simulink model "M10B39_V2"  (R2025a)
settings: Solver=ode23tb  StartTime=0.0  StopTime=1000  FixedStep=0.001  RelTol=1e-3  EnableMultiTasking=on
InitFcn:
  | clear;
  | initAll_V2;
  | %set_param('M10B39/Python2Sim','value','zeros(1,16)');
values from neighbouring files (symbols this model uses):
  acom = 100    [initAll.m]    (also in initAll_V2.m)
  bcom = 50    [initAll.m]    (also in initAll_V2.m)
  commun = 0*commun    [initAll.m]    (also in initAll_V2.m)
  DataDelay = 0.0*DataDelay    [initAll.m]    (also in initAll_V2.m)
  fB = 50    [initAll.m]    (also in initAll_V2.m)
  Geninit = Generator_init(opdata,SynMach_in_gidx)    [initAll.m]    (also in initAll_V2.m)
  lam = 100    [initAll.m]    (also in initAll_V2.m)
  loadnode = 31    [initAll_V2.m]
  loadsize = 16.2714    [initAll_V2.m]
  SgridB = 100    [initAll.m]    (also in initAll_V2.m)
  wB = 2*pi*fB    (= 314.159265359)    [initAll.m]    (also in initAll_V2.m)
undefined symbols (not defined in the file or in its folder): AVm0, c1, c2, c3, c4, c5, c6, cp_nom, ESinit, lambda_nom, P_wind_base, Pelec_base, Pnom, Windinit, YY_load
libraries: spsBistableLib x13, simulink_extras x5, powerlib_meascontrol x2, simulink x1
(part 4 of 11)

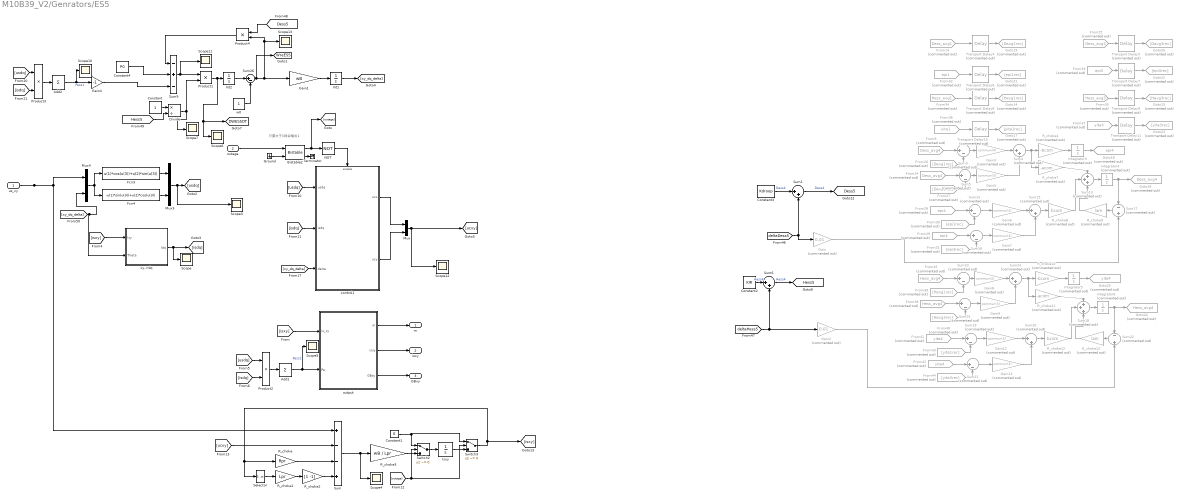
== system M10B39_V2/Genrators/ES5 ==
  note: 只要大于0就会输出1
  us_xy : Inport
  outage : Inport  Port=2
  " control1" : Subsystem
  Add1 : Sum  Inputs=+
  Add2 : Sum  Inputs=+
  Bistable2 : spsBistableLib/Bistable  Qpriority=Set  ic=0  Ts=0
      settings: LibrarySourceBlock=sps_lib/Control/Bistable
  Constant : Constant
  Constant1 : Constant  Value=0
  Constant2 : Constant  Value=KIR
  Constant3 : Constant  Value=Kdroop
  Constant4 : Constant  Value=P0
  Divide : Product  Inputs=*/
  Fcn3 : Fcn  Expr=u(1)*cos(u(3))+u(2)*sin(u(3))
  Fcn4 : Fcn  Expr=-u(1)*sin(u(3))+u(2)*cos(u(3))
  From14 : From  Commented=on  GotoTag=Dess_avg1  TagVisibility=global
  From24 : From  Commented=on  GotoTag=Dess_avg4  TagVisibility=global
  From25 : From  Commented=on  GotoTag=Dess_avg3  TagVisibility=global
  From26 : From  Commented=on  GotoTag=Davg1rec
  From27 : From  Commented=on  GotoTag=Davg3rec
  From28 : From  Commented=on  GotoTag=epi4  TagVisibility=global
  From29 : From  Commented=on  GotoTag=epi4  TagVisibility=global
  From30 : From  Commented=on  GotoTag=epi1rec
  From31 : From  Commented=on  GotoTag=epi3rec
  From32 : From  Commented=on  GotoTag=epi1  TagVisibility=global
  From33 : From  Commented=on  GotoTag=epi3  TagVisibility=global
  From34 : From  Commented=on  GotoTag=Hess_avg1  TagVisibility=global
  From35 : From  Commented=on  GotoTag=Hess_avg3  TagVisibility=global
  From36 : From  Commented=on  GotoTag=yita1  TagVisibility=global
  From37 : From  Commented=on  GotoTag=yita3  TagVisibility=global
  From38 : From  Commented=on  GotoTag=Hess_avg4  TagVisibility=global
  From39 : From  Commented=on  GotoTag=Havg1rec
  From40 : From  Commented=on  GotoTag=Havg3rec
  From41 : From  Commented=on  GotoTag=yita4  TagVisibility=global
  From42 : From  Commented=on  GotoTag=yita4  TagVisibility=global
  From43 : From  Commented=on  GotoTag=yita1rec
  From44 : From  Commented=on  GotoTag=yita3rec
  From45 : From  Commented=on  GotoTag=Hess_avg4  TagVisibility=global
  From9 : From  Commented=on  GotoTag=Dess_avg4  TagVisibility=global
  Gain : Gain  Commented=on  Gain=0.01
  Gain1 : Gain  Gain=wB  SaturateOnIntegerOverflow=on  OutDataTypeStr=Inherit: Same as input  ParamDataTypeStr=Inherit: Same as input
  Gain{3,6,8,12} (4 alike) : Gain  Commented=on  Gain=commun(4)
  Gain{5,7,9,13} (4 alike) : Gain  Commented=on  Gain=commun(3)
  Gain2 : Gain  Commented=on  Gain=0.01
  Gain4 : Gain  Gain=-1
  Goto14 : Goto  Commented=on  GotoTag=Havg1rec
  Goto15 : Goto  Commented=on  GotoTag=Havg3rec
  Goto16 : Goto  Commented=on  GotoTag=Dess_avg4  TagVisibility=global
  Goto17 : Goto  Commented=on  GotoTag=yita1rec
  Goto18 : Goto  Commented=on  GotoTag=epi4  TagVisibility=global
  Goto19 : Goto  Commented=on  GotoTag=Davg1rec
  Goto20 : Goto  Commented=on  GotoTag=Davg3rec
  Goto21 : Goto  Commented=on  GotoTag=epi1rec
  Goto22 : Goto  Commented=on  GotoTag=epi3rec
  Goto23 : Goto  Commented=on  GotoTag=yita3rec
  Goto24 : Goto  Commented=on  GotoTag=Hess_avg4  TagVisibility=global
  Goto25 : Goto  Commented=on  GotoTag=yita4  TagVisibility=global
  Ground : Ground
  Int1 : Integrator  InitialCondition=Dels_hvdc
  Int2 : Integrator  InitialCondition=1
  Integrator{3..6} (4 alike) : Integrator  Commented=on
  Isxy : Integrator  InitialCondition=[Is_xA_0 Is_yA_0]
  Mux : Mux  Inputs=2
  Mux3 : Mux  Inputs=2
  Mux4 : Mux  Inputs=2
  NOT : Logic  Operator=NOT  AllPortsSameDT=off  OutDataTypeStr=boolean
  Product1 : Product
  Product2 : Product  RndMeth=Zero
  Product3 : Product  RndMeth=Zero
  Product4 : Product
  R_choke : Gain  Gain=Rpr  SaturateOnIntegerOverflow=on  OutDataTypeStr=Inherit: Same as input  ParamDataTypeStr=Inherit: Same as input
  R_choke1 : Gain  Gain=Lpr  SaturateOnIntegerOverflow=on  OutDataTypeStr=Inherit: Same as input  ParamDataTypeStr=Inherit: Same as input
  R_choke10 : Gain  Commented=on  Gain=-bcom  SaturateOnIntegerOverflow=on  OutDataTypeStr=Inherit: Same as input  ParamDataTypeStr=Inherit: Same as input
  R_choke11 : Gain  Commented=on  Gain=-acom  SaturateOnIntegerOverflow=on  OutDataTypeStr=Inherit: Same as input  ParamDataTypeStr=Inherit: Same as input
  R_choke12 : Gain  Commented=on  Gain=bcom  SaturateOnIntegerOverflow=on  OutDataTypeStr=Inherit: Same as input  ParamDataTypeStr=Inherit: Same as input
  R_choke13 : Gain  Commented=on  Gain=lam  SaturateOnIntegerOverflow=on  OutDataTypeStr=Inherit: Same as input  ParamDataTypeStr=Inherit: Same as input
  R_choke2 : Gain  Gain=[1 -1]  SaturateOnIntegerOverflow=on  OutDataTypeStr=Inherit: Same as input  ParamDataTypeStr=Inherit: Same as input
  R_choke3 : Gain  Gain=wB / Lpr  SaturateOnIntegerOverflow=on  OutDataTypeStr=Inherit: Same as input  ParamDataTypeStr=Inherit: Same as input
  R_choke4 : Gain  Commented=on  Gain=-bcom  SaturateOnIntegerOverflow=on  OutDataTypeStr=Inherit: Same as input  ParamDataTypeStr=Inherit: Same as input
  R_choke7 : Gain  Commented=on  Gain=-acom  SaturateOnIntegerOverflow=on  OutDataTypeStr=Inherit: Same as input  ParamDataTypeStr=Inherit: Same as input
  R_choke8 : Gain  Commented=on  Gain=bcom  SaturateOnIntegerOverflow=on  OutDataTypeStr=Inherit: Same as input  ParamDataTypeStr=Inherit: Same as input
  R_choke9 : Gain  Commented=on  Gain=lam  SaturateOnIntegerOverflow=on  OutDataTypeStr=Inherit: Same as input  ParamDataTypeStr=Inherit: Same as input
  Scope{,3..7,10..13} (10 alike) : Scope
      Scope settings: ActiveDisplayYMinimum=-0.0194  ActiveDisplayYMaximum=0.04689
      Scope10 settings: ActiveDisplayYMinimum=-6.46308  ActiveDisplayYMaximum=-6.45084
      Scope11 settings: ActiveDisplayYMinimum=-0.1125  ActiveDisplayYMaximum=0.0125  DataLoggingVariableName=ScopeData2
      Scope12 settings: ActiveDisplayYMinimum=0.46883  ActiveDisplayYMaximum=1.25548  DataLoggingVariableName=ScopeData3
      Scope13 settings: ActiveDisplayYMinimum=-0.00656  ActiveDisplayYMaximum=0.05904  DataLoggingVariableName=ScopeData4
      Scope3 settings: ActiveDisplayYMinimum=-0.12696  ActiveDisplayYMaximum=1.14248
      Scope4 settings: ActiveDisplayYMinimum=-2.8E-5  ActiveDisplayYMaximum=2.4E-5  DataLoggingVariableName=ScopeData5
      Scope5 settings: ActiveDisplayYMinimum=-0.00823  ActiveDisplayYMaximum=0.07404  DataLoggingVariableName=ScopeData7
      Scope6 settings: ActiveDisplayYMinimum=-4.9E-5  ActiveDisplayYMaximum=-0  DataLoggingVariableName=ScopeData4
      Scope7 settings: ActiveDisplayYMinimum=0.01956  ActiveDisplayYMaximum=0.02005  DataLoggingVariableName=ScopeData14
  Selector : Selector  InputPortWidth=2  IndexOptions=Index vector (dialog)  Indices=[2 1]  OutputSizes=1
  Sum : Sum  Inputs=+--+  SaturateOnIntegerOverflow=on
  Sum1 : Sum  Inputs=|++  SaturateOnIntegerOverflow=on
  Sum13 : Sum  Commented=on  Inputs=+++  SaturateOnIntegerOverflow=on
  Sum{3,5,14,16,19,21,23,25} (8 alike) : Sum  Commented=on  Inputs=|+-  SaturateOnIntegerOverflow=on
  Sum{4,15,20,24} (4 alike) : Sum  Commented=on  Inputs=|++  SaturateOnIntegerOverflow=on
  Sum17 : Sum  Commented=on  Inputs=-+  SaturateOnIntegerOverflow=on
  Sum18 : Sum  Commented=on  Inputs=+++  SaturateOnIntegerOverflow=on
  Sum22 : Sum  Commented=on  Inputs=-+  SaturateOnIntegerOverflow=on
  Sum26 : Sum  Inputs=|+-  SaturateOnIntegerOverflow=on
  Sum6 : Sum  Inputs=|++  SaturateOnIntegerOverflow=on
  Sum9 : Sum  Inputs=-+-  SaturateOnIntegerOverflow=on
  Switch2 : Switch  Criteria=u2 ~= 0  Threshold=0.5  InputSameDT=off
  Switch3 : Switch  Criteria=u2 ~= 0  Threshold=0.5  InputSameDT=off
  Terminator : Terminator
  Transport Delay{4,6,8,10} (4 alike) : TransportDelay  Commented=on  DelayTime=DataDelay(1,1)
  Transport Delay{5,7,9,11} (4 alike) : TransportDelay  Commented=on  DelayTime=DataDelay(3,2)
  output : Subsystem
  w0 : Constant
  xy->dq : Subsystem
  m : Outport
  isxy : Outport  Port=2
  GBxy : Outport  Port=3
  tag scope: DWES5DT=global, Dess5=global, Hess5=global, WreES5=global
  wires:
  Selector/1 -> R_choke1/1
  Sum/1 -> Scope4/1, R_choke3/1
  R_choke3/1 -> Switch2/3
  Ground/1 -> Bistable2/2
  R_choke2/1 -> Sum/4
  R_choke/1 -> Sum/3
  [ucxy] -> Sum/2
  output/1(m) -> m/1
  NOT/1 -> " control1"/Enable
  R_choke1/1 -> R_choke2/1
  Bistable2/1 -> NOT/1, [outage]
  Isxy/1 -> Switch3/3
  [isxy] -> xy->dq/1(Ixy)
  [isxy] -> output/1(is_xy)
  output/2(isxy) -> isxy/1
  [xy_dq_delta] -> " control1"/3(delta)
  xy->dq/1(Idq) -> [isdq], Scope/1
  Bistable2/2 -> Terminator/1
  outage/1 -> Bistable2/1
  [outage] -> Switch2/2, Switch3/2
  [isdq] -> " control1"/2(isdq)
  " control1"/1(ucx) -> Mux/1
  Switch2/1 -> Isxy/1
  Switch3/1 -> R_choke/1, Selector/1, [isxy]
  Mux/1 -> Scope12/1, [ucxy]
  [usdq] -> " control1"/1(usdq)
  output/3(GBxy) -> GBxy/1
  Constant1/1 -> Switch2/1, Switch3/1
  " control1"/2(ucy) -> Mux/2
  [usdq] -> Product2/1
  Add1/1 -> output/2(Pe), Scope5/1  "Pess1"
  Product2/1 -> Add1/1
  [isdq] -> Product2/2
  Product1/1 -> Scope6/1, [DWES5DT], Int2/1
  Sum26/1 -> [WreES5], Gain1/1, Scope13/1, Product4/2
  Int2/1 -> Sum26/1
  w0/1 -> Sum26/2
  Sum9/1 -> Product1/1, Scope11/1
  Constant/1 -> Divide/1
  Divide/1 -> Product1/2, Scope7/1
  [Hess5] -> Divide/2
  us_xy/1 -> Mux4/1, Sum/1
  Fcn3/1 -> Mux3/1
  Fcn4/1 -> Mux3/2
  Mux4/1 -> Fcn3/1, Fcn4/1
  [xy_dq_delta] -> Mux4/2, xy->dq/2(Theta)
  Mux3/1 -> Scope3/1, [usdq]
  Gain4/1 -> Sum9/3
  Constant4/1 -> Sum9/2
  Product4/1 -> Sum9/1
  Int1/1 -> [xy_dq_delta]
  Add2/1 -> Gain4/1, Scope10/1  "Pess1"
  [usdq] -> Product3/1
  [isdq] -> Product3/2
  Product3/1 -> Add2/1
  [Dess5] -> Product4/1
  Gain1/1 -> Int1/1
  Integrator4/1 -> Sum17/1, Goto16/1
  From30/1 -> Sum14/2
  From31/1 -> Sum16/2
  [deltaDess5] -> Sum1/2, Gain/1
  R_choke9/1 -> Sum13/3
  Sum20/1 -> R_choke12/1
  Constant2/1 -> Sum6/1  "Hess4"
  From29/1 -> Sum16/1
  Constant3/1 -> Sum1/1  "Dess4"
  Sum24/1 -> R_choke11/1, R_choke10/1
  Integrator3/1 -> Goto18/1
  Sum15/1 -> R_choke8/1
  From26/1 -> Sum3/2
  Transport Delay4/1 -> Goto19/1
  Transport Delay5/1 -> Goto20/1
  R_choke4/1 -> Integrator3/1
  Transport Delay7/1 -> Goto22/1
  From39/1 -> Sum23/2
  Transport Delay8/1 -> Goto14/1
  Sum17/1 -> R_choke9/1
  Transport Delay6/1 -> Goto21/1
  Sum13/1 -> Integrator4/1
  Transport Delay10/1 -> Goto17/1
  From40/1 -> Sum25/2
  Transport Delay9/1 -> Goto15/1
  Transport Delay11/1 -> Goto23/1
  From45/1 -> Sum23/1
  R_choke10/1 -> Integrator5/1
  From42/1 -> Sum21/1
  R_choke8/1 -> Sum13/2
  From28/1 -> Sum14/1
  From24/1 -> Sum5/1
  R_choke7/1 -> Sum13/1
  Sum18/1 -> Integrator6/1
  R_choke12/1 -> Sum18/2
  From38/1 -> Sum25/1
  Sum22/1 -> R_choke13/1
  R_choke13/1 -> Sum18/3
  From41/1 -> Sum19/1
  Sum4/1 -> R_choke7/1, R_choke4/1
  From44/1 -> Sum21/2
  R_choke11/1 -> Sum18/1
  From27/1 -> Sum5/2
  From9/1 -> Sum3/1
  Integrator6/1 -> Sum22/1, Goto24/1
  From43/1 -> Sum19/2
  Integrator5/1 -> Goto25/1
  [deltaHess5] -> Gain2/1, Sum6/2
  Gain/1 -> Sum17/2
  Gain2/1 -> Sum22/2
  From14/1 -> Transport Delay4/1
  From32/1 -> Transport Delay6/1
  From34/1 -> Transport Delay8/1
  From36/1 -> Transport Delay10/1
  From25/1 -> Transport Delay5/1
  From33/1 -> Transport Delay7/1
  From35/1 -> Transport Delay9/1
  From37/1 -> Transport Delay11/1
  Sum3/1 -> Gain3/1
  Gain3/1 -> Sum4/1
  Sum5/1 -> Gain5/1
  Gain5/1 -> Sum4/2
  Gain6/1 -> Sum15/1
  Sum14/1 -> Gain6/1
  Sum16/1 -> Gain7/1
  Gain7/1 -> Sum15/2
  Sum23/1 -> Gain8/1
  Gain8/1 -> Sum24/1
  Gain9/1 -> Sum24/2
  Sum25/1 -> Gain9/1
  Gain12/1 -> Sum20/1
  Sum19/1 -> Gain12/1
  Sum21/1 -> Gain13/1
  Gain13/1 -> Sum20/2
  Sum1/1 -> [Dess5]  "Dess4"
  Sum6/1 -> [Hess5]  "Hess4"

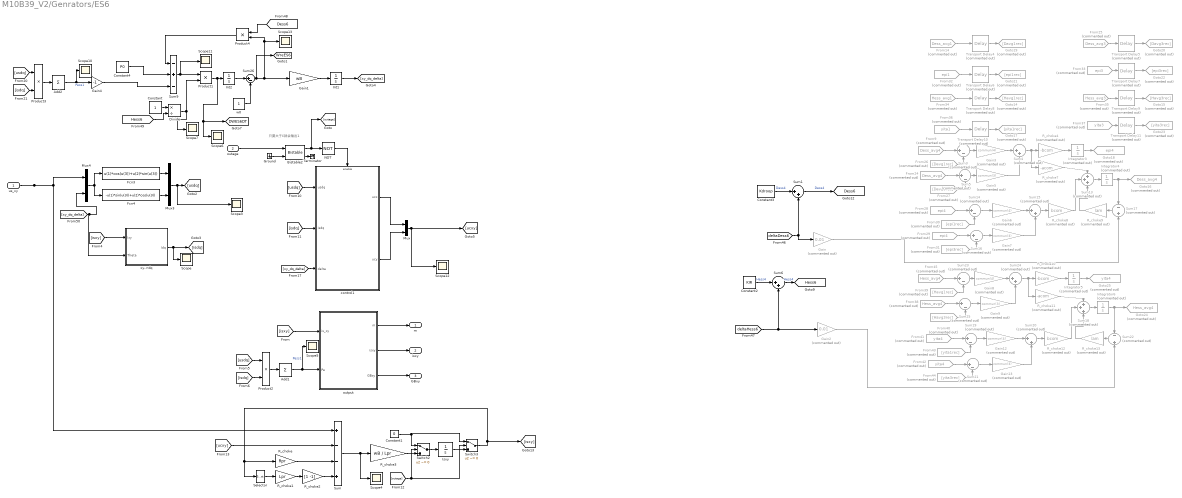
== system M10B39_V2/Genrators/ES6 ==
  note: 只要大于0就会输出1
  us_xy : Inport
  outage : Inport  Port=2
  " control1" : Subsystem
  Add1 : Sum  Inputs=+
  Add2 : Sum  Inputs=+
  Bistable2 : spsBistableLib/Bistable  Qpriority=Set  ic=0  Ts=0
      settings: LibrarySourceBlock=sps_lib/Control/Bistable
  Constant : Constant
  Constant1 : Constant  Value=0
  Constant2 : Constant  Value=KIR
  Constant3 : Constant  Value=Kdroop
  Constant4 : Constant  Value=P0
  Divide : Product  Inputs=*/
  Fcn3 : Fcn  Expr=u(1)*cos(u(3))+u(2)*sin(u(3))
  Fcn4 : Fcn  Expr=-u(1)*sin(u(3))+u(2)*cos(u(3))
  From14 : From  Commented=on  GotoTag=Dess_avg1  TagVisibility=global
  From24 : From  Commented=on  GotoTag=Dess_avg4  TagVisibility=global
  From25 : From  Commented=on  GotoTag=Dess_avg3  TagVisibility=global
  From26 : From  Commented=on  GotoTag=Davg1rec
  From27 : From  Commented=on  GotoTag=Davg3rec
  From28 : From  Commented=on  GotoTag=epi4  TagVisibility=global
  From29 : From  Commented=on  GotoTag=epi4  TagVisibility=global
  From30 : From  Commented=on  GotoTag=epi1rec
  From31 : From  Commented=on  GotoTag=epi3rec
  From32 : From  Commented=on  GotoTag=epi1  TagVisibility=global
  From33 : From  Commented=on  GotoTag=epi3  TagVisibility=global
  From34 : From  Commented=on  GotoTag=Hess_avg1  TagVisibility=global
  From35 : From  Commented=on  GotoTag=Hess_avg3  TagVisibility=global
  From36 : From  Commented=on  GotoTag=yita1  TagVisibility=global
  From37 : From  Commented=on  GotoTag=yita3  TagVisibility=global
  From38 : From  Commented=on  GotoTag=Hess_avg4  TagVisibility=global
  From39 : From  Commented=on  GotoTag=Havg1rec
  From40 : From  Commented=on  GotoTag=Havg3rec
  From41 : From  Commented=on  GotoTag=yita4  TagVisibility=global
  From42 : From  Commented=on  GotoTag=yita4  TagVisibility=global
  From43 : From  Commented=on  GotoTag=yita1rec
  From44 : From  Commented=on  GotoTag=yita3rec
  From45 : From  Commented=on  GotoTag=Hess_avg4  TagVisibility=global
  From9 : From  Commented=on  GotoTag=Dess_avg4  TagVisibility=global
  Gain : Gain  Commented=on  Gain=0.01
  Gain1 : Gain  Gain=wB  SaturateOnIntegerOverflow=on  OutDataTypeStr=Inherit: Same as input  ParamDataTypeStr=Inherit: Same as input
  Gain{3,6,8,12} (4 alike) : Gain  Commented=on  Gain=commun(4)
  Gain{5,7,9,13} (4 alike) : Gain  Commented=on  Gain=commun(3)
  Gain2 : Gain  Commented=on  Gain=0.01
  Gain4 : Gain  Gain=-1
  Goto14 : Goto  Commented=on  GotoTag=Havg1rec
  Goto15 : Goto  Commented=on  GotoTag=Havg3rec
  Goto16 : Goto  Commented=on  GotoTag=Dess_avg4  TagVisibility=global
  Goto17 : Goto  Commented=on  GotoTag=yita1rec
  Goto18 : Goto  Commented=on  GotoTag=epi4  TagVisibility=global
  Goto19 : Goto  Commented=on  GotoTag=Davg1rec
  Goto20 : Goto  Commented=on  GotoTag=Davg3rec
  Goto21 : Goto  Commented=on  GotoTag=epi1rec
  Goto22 : Goto  Commented=on  GotoTag=epi3rec
  Goto23 : Goto  Commented=on  GotoTag=yita3rec
  Goto24 : Goto  Commented=on  GotoTag=Hess_avg4  TagVisibility=global
  Goto25 : Goto  Commented=on  GotoTag=yita4  TagVisibility=global
  Ground : Ground
  Int1 : Integrator  InitialCondition=Dels_hvdc
  Int2 : Integrator  InitialCondition=1
  Integrator{3..6} (4 alike) : Integrator  Commented=on
  Isxy : Integrator  InitialCondition=[Is_xA_0 Is_yA_0]
  Mux : Mux  Inputs=2
  Mux3 : Mux  Inputs=2
  Mux4 : Mux  Inputs=2
  NOT : Logic  Operator=NOT  AllPortsSameDT=off  OutDataTypeStr=boolean
  Product1 : Product
  Product2 : Product  RndMeth=Zero
  Product3 : Product  RndMeth=Zero
  Product4 : Product
  R_choke : Gain  Gain=Rpr  SaturateOnIntegerOverflow=on  OutDataTypeStr=Inherit: Same as input  ParamDataTypeStr=Inherit: Same as input
  R_choke1 : Gain  Gain=Lpr  SaturateOnIntegerOverflow=on  OutDataTypeStr=Inherit: Same as input  ParamDataTypeStr=Inherit: Same as input
  R_choke10 : Gain  Commented=on  Gain=-bcom  SaturateOnIntegerOverflow=on  OutDataTypeStr=Inherit: Same as input  ParamDataTypeStr=Inherit: Same as input
  R_choke11 : Gain  Commented=on  Gain=-acom  SaturateOnIntegerOverflow=on  OutDataTypeStr=Inherit: Same as input  ParamDataTypeStr=Inherit: Same as input
  R_choke12 : Gain  Commented=on  Gain=bcom  SaturateOnIntegerOverflow=on  OutDataTypeStr=Inherit: Same as input  ParamDataTypeStr=Inherit: Same as input
  R_choke13 : Gain  Commented=on  Gain=lam  SaturateOnIntegerOverflow=on  OutDataTypeStr=Inherit: Same as input  ParamDataTypeStr=Inherit: Same as input
  R_choke2 : Gain  Gain=[1 -1]  SaturateOnIntegerOverflow=on  OutDataTypeStr=Inherit: Same as input  ParamDataTypeStr=Inherit: Same as input
  R_choke3 : Gain  Gain=wB / Lpr  SaturateOnIntegerOverflow=on  OutDataTypeStr=Inherit: Same as input  ParamDataTypeStr=Inherit: Same as input
  R_choke4 : Gain  Commented=on  Gain=-bcom  SaturateOnIntegerOverflow=on  OutDataTypeStr=Inherit: Same as input  ParamDataTypeStr=Inherit: Same as input
  R_choke7 : Gain  Commented=on  Gain=-acom  SaturateOnIntegerOverflow=on  OutDataTypeStr=Inherit: Same as input  ParamDataTypeStr=Inherit: Same as input
  R_choke8 : Gain  Commented=on  Gain=bcom  SaturateOnIntegerOverflow=on  OutDataTypeStr=Inherit: Same as input  ParamDataTypeStr=Inherit: Same as input
  R_choke9 : Gain  Commented=on  Gain=lam  SaturateOnIntegerOverflow=on  OutDataTypeStr=Inherit: Same as input  ParamDataTypeStr=Inherit: Same as input
  Scope{,3..7,10..13} (10 alike) : Scope
      Scope settings: ActiveDisplayYMinimum=-0.0194  ActiveDisplayYMaximum=0.04689
      Scope10 settings: ActiveDisplayYMinimum=-6.46308  ActiveDisplayYMaximum=-6.45084
      Scope11 settings: ActiveDisplayYMinimum=-0.1125  ActiveDisplayYMaximum=0.0125  DataLoggingVariableName=ScopeData2
      Scope12 settings: ActiveDisplayYMinimum=0.46883  ActiveDisplayYMaximum=1.25548  DataLoggingVariableName=ScopeData3
      Scope13 settings: ActiveDisplayYMinimum=-0.00656  ActiveDisplayYMaximum=0.05904  DataLoggingVariableName=ScopeData4
      Scope3 settings: ActiveDisplayYMinimum=-0.12696  ActiveDisplayYMaximum=1.14248
      Scope4 settings: ActiveDisplayYMinimum=-2.8E-5  ActiveDisplayYMaximum=2.4E-5  DataLoggingVariableName=ScopeData5
      Scope5 settings: ActiveDisplayYMinimum=-0.00823  ActiveDisplayYMaximum=0.07404  DataLoggingVariableName=ScopeData7
      Scope6 settings: ActiveDisplayYMinimum=-4.9E-5  ActiveDisplayYMaximum=-0  DataLoggingVariableName=ScopeData4
      Scope7 settings: ActiveDisplayYMinimum=0.9  ActiveDisplayYMaximum=1.1  DataLoggingVariableName=ScopeData14
  Selector : Selector  InputPortWidth=2  IndexOptions=Index vector (dialog)  Indices=[2 1]  OutputSizes=1
  Sum : Sum  Inputs=+--+  SaturateOnIntegerOverflow=on
  Sum1 : Sum  Inputs=|++  SaturateOnIntegerOverflow=on
  Sum13 : Sum  Commented=on  Inputs=+++  SaturateOnIntegerOverflow=on
  Sum{3,5,14,16,19,21,23,25} (8 alike) : Sum  Commented=on  Inputs=|+-  SaturateOnIntegerOverflow=on
  Sum{4,15,20,24} (4 alike) : Sum  Commented=on  Inputs=|++  SaturateOnIntegerOverflow=on
  Sum17 : Sum  Commented=on  Inputs=-+  SaturateOnIntegerOverflow=on
  Sum18 : Sum  Commented=on  Inputs=+++  SaturateOnIntegerOverflow=on
  Sum22 : Sum  Commented=on  Inputs=-+  SaturateOnIntegerOverflow=on
  Sum26 : Sum  Inputs=|+-  SaturateOnIntegerOverflow=on
  Sum6 : Sum  Inputs=|++  SaturateOnIntegerOverflow=on
  Sum9 : Sum  Inputs=-+-  SaturateOnIntegerOverflow=on
  Switch2 : Switch  Criteria=u2 ~= 0  Threshold=0.5  InputSameDT=off
  Switch3 : Switch  Criteria=u2 ~= 0  Threshold=0.5  InputSameDT=off
  Terminator : Terminator
  Transport Delay{4,6,8,10} (4 alike) : TransportDelay  Commented=on  DelayTime=DataDelay(1,1)
  Transport Delay{5,7,9,11} (4 alike) : TransportDelay  Commented=on  DelayTime=DataDelay(3,2)
  output : Subsystem
  w0 : Constant
  xy->dq : Subsystem
  m : Outport
  isxy : Outport  Port=2
  GBxy : Outport  Port=3
  tag scope: DWES6DT=global, Dess6=global, Hess6=global, WreES6=global
  wires:
  Gain13/1 -> Sum20/2
  Sum21/1 -> Gain13/1
  Sum19/1 -> Gain12/1
  Gain12/1 -> Sum20/1
  Sum25/1 -> Gain9/1
  Gain9/1 -> Sum24/2
  Gain8/1 -> Sum24/1
  Sum23/1 -> Gain8/1
  Gain7/1 -> Sum15/2
  Sum16/1 -> Gain7/1
  Sum14/1 -> Gain6/1
  Gain6/1 -> Sum15/1
  Gain5/1 -> Sum4/2
  Sum5/1 -> Gain5/1
  Gain3/1 -> Sum4/1
  Sum3/1 -> Gain3/1
  From37/1 -> Transport Delay11/1
  From35/1 -> Transport Delay9/1
  From33/1 -> Transport Delay7/1
  From25/1 -> Transport Delay5/1
  From36/1 -> Transport Delay10/1
  From34/1 -> Transport Delay8/1
  From32/1 -> Transport Delay6/1
  From14/1 -> Transport Delay4/1
  Gain2/1 -> Sum22/2
  Gain/1 -> Sum17/2
  [deltaHess6] -> Sum6/2, Gain2/1
  Integrator5/1 -> Goto25/1
  From43/1 -> Sum19/2
  Integrator6/1 -> Goto24/1, Sum22/1
  From9/1 -> Sum3/1
  From27/1 -> Sum5/2
  R_choke11/1 -> Sum18/1
  From44/1 -> Sum21/2
  Sum4/1 -> R_choke4/1, R_choke7/1
  From41/1 -> Sum19/1
  R_choke13/1 -> Sum18/3
  Sum22/1 -> R_choke13/1
  From38/1 -> Sum25/1
  R_choke12/1 -> Sum18/2
  Sum18/1 -> Integrator6/1
  R_choke7/1 -> Sum13/1
  From24/1 -> Sum5/1
  From28/1 -> Sum14/1
  R_choke8/1 -> Sum13/2
  From42/1 -> Sum21/1
  R_choke10/1 -> Integrator5/1
  From45/1 -> Sum23/1
  Transport Delay11/1 -> Goto23/1
  Transport Delay9/1 -> Goto15/1
  From40/1 -> Sum25/2
  Transport Delay10/1 -> Goto17/1
  Sum13/1 -> Integrator4/1
  Transport Delay6/1 -> Goto21/1
  Sum17/1 -> R_choke9/1
  Transport Delay8/1 -> Goto14/1
  From39/1 -> Sum23/2
  Transport Delay7/1 -> Goto22/1
  R_choke4/1 -> Integrator3/1
  Transport Delay5/1 -> Goto20/1
  Transport Delay4/1 -> Goto19/1
  From26/1 -> Sum3/2
  Sum15/1 -> R_choke8/1
  Integrator3/1 -> Goto18/1
  Sum24/1 -> R_choke10/1, R_choke11/1
  Constant3/1 -> Sum1/1  "Dess4"
  From29/1 -> Sum16/1
  Constant2/1 -> Sum6/1  "Hess4"
  Sum20/1 -> R_choke12/1
  R_choke9/1 -> Sum13/3
  [deltaDess6] -> Gain/1, Sum1/2
  From31/1 -> Sum16/2
  From30/1 -> Sum14/2
  Integrator4/1 -> Goto16/1, Sum17/1
  Gain1/1 -> Int1/1
  [Dess6] -> Product4/1
  Product3/1 -> Add2/1
  [isdq] -> Product3/2
  [usdq] -> Product3/1
  Add2/1 -> Scope10/1, Gain4/1  "Pess1"
  Int1/1 -> [xy_dq_delta]
  Product4/1 -> Sum9/1
  Constant4/1 -> Sum9/2
  Gain4/1 -> Sum9/3
  Mux3/1 -> [usdq], Scope3/1
  [xy_dq_delta] -> xy->dq/2(Theta), Mux4/2
  Mux4/1 -> Fcn4/1, Fcn3/1
  Fcn4/1 -> Mux3/2
  Fcn3/1 -> Mux3/1
  us_xy/1 -> Sum/1, Mux4/1
  [Hess6] -> Divide/2
  Divide/1 -> Scope7/1, Product1/2
  Constant/1 -> Divide/1
  Sum9/1 -> Scope11/1, Product1/1
  w0/1 -> Sum26/2
  Int2/1 -> Sum26/1
  Sum26/1 -> Product4/2, Scope13/1, Gain1/1, [WreES6]
  Product1/1 -> Int2/1, [DWES6DT], Scope6/1
  [isdq] -> Product2/2
  Product2/1 -> Add1/1
  Add1/1 -> output/2(Pe), Scope5/1  "Pess1"
  [usdq] -> Product2/1
  " control1"/2(ucy) -> Mux/2
  Constant1/1 -> Switch3/1, Switch2/1
  output/3(GBxy) -> GBxy/1
  [usdq] -> " control1"/1(usdq)
  Mux/1 -> [ucxy], Scope12/1
  Switch3/1 -> [isxy], Selector/1, R_choke/1
  Switch2/1 -> Isxy/1
  " control1"/1(ucx) -> Mux/1
  [isdq] -> " control1"/2(isdq)
  [outage] -> Switch3/2, Switch2/2
  outage/1 -> Bistable2/1
  Bistable2/2 -> Terminator/1
  xy->dq/1(Idq) -> Scope/1, [isdq]
  [xy_dq_delta] -> " control1"/3(delta)
  output/2(isxy) -> isxy/1
  [isxy] -> output/1(is_xy)
  [isxy] -> xy->dq/1(Ixy)
  Isxy/1 -> Switch3/3
  Bistable2/1 -> [outage], NOT/1
  R_choke1/1 -> R_choke2/1
  NOT/1 -> " control1"/Enable
  output/1(m) -> m/1
  [ucxy] -> Sum/2
  R_choke/1 -> Sum/3
  R_choke2/1 -> Sum/4
  Ground/1 -> Bistable2/2
  R_choke3/1 -> Switch2/3
  Sum/1 -> R_choke3/1, Scope4/1
  Selector/1 -> R_choke1/1
  Sum1/1 -> [Dess6]  "Dess4"
  Sum6/1 -> [Hess6]  "Hess4"

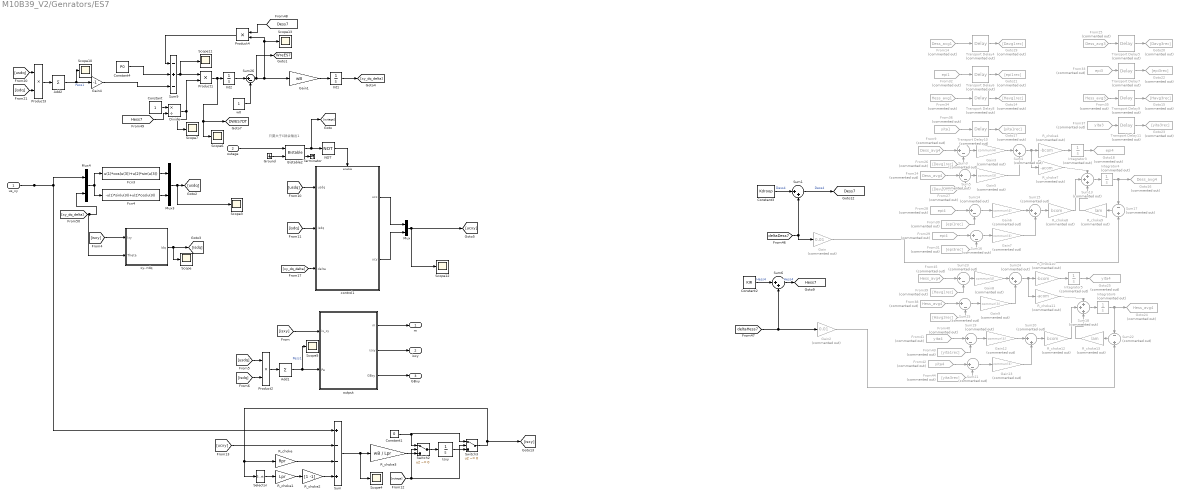
== system M10B39_V2/Genrators/ES7 ==
  note: 只要大于0就会输出1
  us_xy : Inport
  outage : Inport  Port=2
  " control1" : Subsystem
  Add1 : Sum  Inputs=+
  Add2 : Sum  Inputs=+
  Bistable2 : spsBistableLib/Bistable  Qpriority=Set  ic=0  Ts=0
      settings: LibrarySourceBlock=sps_lib/Control/Bistable
  Constant : Constant
  Constant1 : Constant  Value=0
  Constant2 : Constant  Value=KIR
  Constant3 : Constant  Value=Kdroop
  Constant4 : Constant  Value=P0
  Divide : Product  Inputs=*/
  Fcn3 : Fcn  Expr=u(1)*cos(u(3))+u(2)*sin(u(3))
  Fcn4 : Fcn  Expr=-u(1)*sin(u(3))+u(2)*cos(u(3))
  From14 : From  Commented=on  GotoTag=Dess_avg1  TagVisibility=global
  From24 : From  Commented=on  GotoTag=Dess_avg4  TagVisibility=global
  From25 : From  Commented=on  GotoTag=Dess_avg3  TagVisibility=global
  From26 : From  Commented=on  GotoTag=Davg1rec
  From27 : From  Commented=on  GotoTag=Davg3rec
  From28 : From  Commented=on  GotoTag=epi4  TagVisibility=global
  From29 : From  Commented=on  GotoTag=epi4  TagVisibility=global
  From30 : From  Commented=on  GotoTag=epi1rec
  From31 : From  Commented=on  GotoTag=epi3rec
  From32 : From  Commented=on  GotoTag=epi1  TagVisibility=global
  From33 : From  Commented=on  GotoTag=epi3  TagVisibility=global
  From34 : From  Commented=on  GotoTag=Hess_avg1  TagVisibility=global
  From35 : From  Commented=on  GotoTag=Hess_avg3  TagVisibility=global
  From36 : From  Commented=on  GotoTag=yita1  TagVisibility=global
  From37 : From  Commented=on  GotoTag=yita3  TagVisibility=global
  From38 : From  Commented=on  GotoTag=Hess_avg4  TagVisibility=global
  From39 : From  Commented=on  GotoTag=Havg1rec
  From40 : From  Commented=on  GotoTag=Havg3rec
  From41 : From  Commented=on  GotoTag=yita4  TagVisibility=global
  From42 : From  Commented=on  GotoTag=yita4  TagVisibility=global
  From43 : From  Commented=on  GotoTag=yita1rec
  From44 : From  Commented=on  GotoTag=yita3rec
  From45 : From  Commented=on  GotoTag=Hess_avg4  TagVisibility=global
  From9 : From  Commented=on  GotoTag=Dess_avg4  TagVisibility=global
  Gain : Gain  Commented=on  Gain=0.01
  Gain1 : Gain  Gain=wB  SaturateOnIntegerOverflow=on  OutDataTypeStr=Inherit: Same as input  ParamDataTypeStr=Inherit: Same as input
  Gain{3,6,8,12} (4 alike) : Gain  Commented=on  Gain=commun(4)
  Gain{5,7,9,13} (4 alike) : Gain  Commented=on  Gain=commun(3)
  Gain2 : Gain  Commented=on  Gain=0.01
  Gain4 : Gain  Gain=-1
  Goto14 : Goto  Commented=on  GotoTag=Havg1rec
  Goto15 : Goto  Commented=on  GotoTag=Havg3rec
  Goto16 : Goto  Commented=on  GotoTag=Dess_avg4  TagVisibility=global
  Goto17 : Goto  Commented=on  GotoTag=yita1rec
  Goto18 : Goto  Commented=on  GotoTag=epi4  TagVisibility=global
  Goto19 : Goto  Commented=on  GotoTag=Davg1rec
  Goto20 : Goto  Commented=on  GotoTag=Davg3rec
  Goto21 : Goto  Commented=on  GotoTag=epi1rec
  Goto22 : Goto  Commented=on  GotoTag=epi3rec
  Goto23 : Goto  Commented=on  GotoTag=yita3rec
  Goto24 : Goto  Commented=on  GotoTag=Hess_avg4  TagVisibility=global
  Goto25 : Goto  Commented=on  GotoTag=yita4  TagVisibility=global
  Ground : Ground
  Int1 : Integrator  InitialCondition=Dels_hvdc
  Int2 : Integrator  InitialCondition=1
  Integrator{3..6} (4 alike) : Integrator  Commented=on
  Isxy : Integrator  InitialCondition=[Is_xA_0 Is_yA_0]
  Mux : Mux  Inputs=2
  Mux3 : Mux  Inputs=2
  Mux4 : Mux  Inputs=2
  NOT : Logic  Operator=NOT  AllPortsSameDT=off  OutDataTypeStr=boolean
  Product1 : Product
  Product2 : Product  RndMeth=Zero
  Product3 : Product  RndMeth=Zero
  Product4 : Product
  R_choke : Gain  Gain=Rpr  SaturateOnIntegerOverflow=on  OutDataTypeStr=Inherit: Same as input  ParamDataTypeStr=Inherit: Same as input
  R_choke1 : Gain  Gain=Lpr  SaturateOnIntegerOverflow=on  OutDataTypeStr=Inherit: Same as input  ParamDataTypeStr=Inherit: Same as input
  R_choke10 : Gain  Commented=on  Gain=-bcom  SaturateOnIntegerOverflow=on  OutDataTypeStr=Inherit: Same as input  ParamDataTypeStr=Inherit: Same as input
  R_choke11 : Gain  Commented=on  Gain=-acom  SaturateOnIntegerOverflow=on  OutDataTypeStr=Inherit: Same as input  ParamDataTypeStr=Inherit: Same as input
  R_choke12 : Gain  Commented=on  Gain=bcom  SaturateOnIntegerOverflow=on  OutDataTypeStr=Inherit: Same as input  ParamDataTypeStr=Inherit: Same as input
  R_choke13 : Gain  Commented=on  Gain=lam  SaturateOnIntegerOverflow=on  OutDataTypeStr=Inherit: Same as input  ParamDataTypeStr=Inherit: Same as input
  R_choke2 : Gain  Gain=[1 -1]  SaturateOnIntegerOverflow=on  OutDataTypeStr=Inherit: Same as input  ParamDataTypeStr=Inherit: Same as input
  R_choke3 : Gain  Gain=wB / Lpr  SaturateOnIntegerOverflow=on  OutDataTypeStr=Inherit: Same as input  ParamDataTypeStr=Inherit: Same as input
  R_choke4 : Gain  Commented=on  Gain=-bcom  SaturateOnIntegerOverflow=on  OutDataTypeStr=Inherit: Same as input  ParamDataTypeStr=Inherit: Same as input
  R_choke7 : Gain  Commented=on  Gain=-acom  SaturateOnIntegerOverflow=on  OutDataTypeStr=Inherit: Same as input  ParamDataTypeStr=Inherit: Same as input
  R_choke8 : Gain  Commented=on  Gain=bcom  SaturateOnIntegerOverflow=on  OutDataTypeStr=Inherit: Same as input  ParamDataTypeStr=Inherit: Same as input
  R_choke9 : Gain  Commented=on  Gain=lam  SaturateOnIntegerOverflow=on  OutDataTypeStr=Inherit: Same as input  ParamDataTypeStr=Inherit: Same as input
  Scope{,3..7,10..13} (10 alike) : Scope
      Scope settings: ActiveDisplayYMinimum=-0.0194  ActiveDisplayYMaximum=0.04689
      Scope10 settings: ActiveDisplayYMinimum=-6.46308  ActiveDisplayYMaximum=-6.45084
      Scope11 settings: ActiveDisplayYMinimum=-0.1125  ActiveDisplayYMaximum=0.0125  DataLoggingVariableName=ScopeData2
      Scope12 settings: ActiveDisplayYMinimum=0.46883  ActiveDisplayYMaximum=1.25548  DataLoggingVariableName=ScopeData3
      Scope13 settings: ActiveDisplayYMinimum=-0.00656  ActiveDisplayYMaximum=0.05904  DataLoggingVariableName=ScopeData4
      Scope3 settings: ActiveDisplayYMinimum=-0.12696  ActiveDisplayYMaximum=1.14248
      Scope4 settings: ActiveDisplayYMinimum=-2.8E-5  ActiveDisplayYMaximum=2.4E-5  DataLoggingVariableName=ScopeData5
      Scope5 settings: ActiveDisplayYMinimum=-0.00823  ActiveDisplayYMaximum=0.07404  DataLoggingVariableName=ScopeData7
      Scope6 settings: ActiveDisplayYMinimum=-4.9E-5  ActiveDisplayYMaximum=-0  DataLoggingVariableName=ScopeData4
      Scope7 settings: ActiveDisplayYMinimum=0.9  ActiveDisplayYMaximum=1.1  DataLoggingVariableName=ScopeData14
  Selector : Selector  InputPortWidth=2  IndexOptions=Index vector (dialog)  Indices=[2 1]  OutputSizes=1
  Sum : Sum  Inputs=+--+  SaturateOnIntegerOverflow=on
  Sum1 : Sum  Inputs=|++  SaturateOnIntegerOverflow=on
  Sum13 : Sum  Commented=on  Inputs=+++  SaturateOnIntegerOverflow=on
  Sum{3,5,14,16,19,21,23,25} (8 alike) : Sum  Commented=on  Inputs=|+-  SaturateOnIntegerOverflow=on
  Sum{4,15,20,24} (4 alike) : Sum  Commented=on  Inputs=|++  SaturateOnIntegerOverflow=on
  Sum17 : Sum  Commented=on  Inputs=-+  SaturateOnIntegerOverflow=on
  Sum18 : Sum  Commented=on  Inputs=+++  SaturateOnIntegerOverflow=on
  Sum22 : Sum  Commented=on  Inputs=-+  SaturateOnIntegerOverflow=on
  Sum26 : Sum  Inputs=|+-  SaturateOnIntegerOverflow=on
  Sum6 : Sum  Inputs=|++  SaturateOnIntegerOverflow=on
  Sum9 : Sum  Inputs=-+-  SaturateOnIntegerOverflow=on
  Switch2 : Switch  Criteria=u2 ~= 0  Threshold=0.5  InputSameDT=off
  Switch3 : Switch  Criteria=u2 ~= 0  Threshold=0.5  InputSameDT=off
  Terminator : Terminator
  Transport Delay{4,6,8,10} (4 alike) : TransportDelay  Commented=on  DelayTime=DataDelay(1,1)
  Transport Delay{5,7,9,11} (4 alike) : TransportDelay  Commented=on  DelayTime=DataDelay(3,2)
  output : Subsystem
  w0 : Constant
  xy->dq : Subsystem
  m : Outport
  isxy : Outport  Port=2
  GBxy : Outport  Port=3
  tag scope: DWES7DT=global, Dess7=global, Hess7=global, WreES7=global
  wires:
  Gain13/1 -> Sum20/2
  Sum21/1 -> Gain13/1
  Sum19/1 -> Gain12/1
  Gain12/1 -> Sum20/1
  Sum25/1 -> Gain9/1
  Gain9/1 -> Sum24/2
  Gain8/1 -> Sum24/1
  Sum23/1 -> Gain8/1
  Gain7/1 -> Sum15/2
  Sum16/1 -> Gain7/1
  Sum14/1 -> Gain6/1
  Gain6/1 -> Sum15/1
  Gain5/1 -> Sum4/2
  Sum5/1 -> Gain5/1
  Gain3/1 -> Sum4/1
  Sum3/1 -> Gain3/1
  From37/1 -> Transport Delay11/1
  From35/1 -> Transport Delay9/1
  From33/1 -> Transport Delay7/1
  From25/1 -> Transport Delay5/1
  From36/1 -> Transport Delay10/1
  From34/1 -> Transport Delay8/1
  From32/1 -> Transport Delay6/1
  From14/1 -> Transport Delay4/1
  Gain2/1 -> Sum22/2
  Gain/1 -> Sum17/2
  [deltaHess7] -> Sum6/2, Gain2/1
  Integrator5/1 -> Goto25/1
  From43/1 -> Sum19/2
  Integrator6/1 -> Goto24/1, Sum22/1
  From9/1 -> Sum3/1
  From27/1 -> Sum5/2
  R_choke11/1 -> Sum18/1
  From44/1 -> Sum21/2
  Sum4/1 -> R_choke4/1, R_choke7/1
  From41/1 -> Sum19/1
  R_choke13/1 -> Sum18/3
  Sum22/1 -> R_choke13/1
  From38/1 -> Sum25/1
  R_choke12/1 -> Sum18/2
  Sum18/1 -> Integrator6/1
  R_choke7/1 -> Sum13/1
  From24/1 -> Sum5/1
  From28/1 -> Sum14/1
  R_choke8/1 -> Sum13/2
  From42/1 -> Sum21/1
  R_choke10/1 -> Integrator5/1
  From45/1 -> Sum23/1
  Transport Delay11/1 -> Goto23/1
  Transport Delay9/1 -> Goto15/1
  From40/1 -> Sum25/2
  Transport Delay10/1 -> Goto17/1
  Sum13/1 -> Integrator4/1
  Transport Delay6/1 -> Goto21/1
  Sum17/1 -> R_choke9/1
  Transport Delay8/1 -> Goto14/1
  From39/1 -> Sum23/2
  Transport Delay7/1 -> Goto22/1
  R_choke4/1 -> Integrator3/1
  Transport Delay5/1 -> Goto20/1
  Transport Delay4/1 -> Goto19/1
  From26/1 -> Sum3/2
  Sum15/1 -> R_choke8/1
  Integrator3/1 -> Goto18/1
  Sum24/1 -> R_choke10/1, R_choke11/1
  Constant3/1 -> Sum1/1  "Dess4"
  From29/1 -> Sum16/1
  Constant2/1 -> Sum6/1  "Hess4"
  Sum20/1 -> R_choke12/1
  R_choke9/1 -> Sum13/3
  [deltaDess7] -> Gain/1, Sum1/2
  From31/1 -> Sum16/2
  From30/1 -> Sum14/2
  Integrator4/1 -> Goto16/1, Sum17/1
  Gain1/1 -> Int1/1
  [Dess7] -> Product4/1
  Product3/1 -> Add2/1
  [isdq] -> Product3/2
  [usdq] -> Product3/1
  Add2/1 -> Scope10/1, Gain4/1  "Pess1"
  Int1/1 -> [xy_dq_delta]
  Product4/1 -> Sum9/1
  Constant4/1 -> Sum9/2
  Gain4/1 -> Sum9/3
  Mux3/1 -> [usdq], Scope3/1
  [xy_dq_delta] -> xy->dq/2(Theta), Mux4/2
  Mux4/1 -> Fcn4/1, Fcn3/1
  Fcn4/1 -> Mux3/2
  Fcn3/1 -> Mux3/1
  us_xy/1 -> Sum/1, Mux4/1
  [Hess7] -> Divide/2
  Divide/1 -> Scope7/1, Product1/2
  Constant/1 -> Divide/1
  Sum9/1 -> Scope11/1, Product1/1
  w0/1 -> Sum26/2
  Int2/1 -> Sum26/1
  Sum26/1 -> Product4/2, Scope13/1, Gain1/1, [WreES7]
  Product1/1 -> Int2/1, [DWES7DT], Scope6/1
  [isdq] -> Product2/2
  Product2/1 -> Add1/1
  Add1/1 -> output/2(Pe), Scope5/1  "Pess1"
  [usdq] -> Product2/1
  " control1"/2(ucy) -> Mux/2
  Constant1/1 -> Switch3/1, Switch2/1
  output/3(GBxy) -> GBxy/1
  [usdq] -> " control1"/1(usdq)
  Mux/1 -> [ucxy], Scope12/1
  Switch3/1 -> [isxy], Selector/1, R_choke/1
  Switch2/1 -> Isxy/1
  " control1"/1(ucx) -> Mux/1
  [isdq] -> " control1"/2(isdq)
  [outage] -> Switch3/2, Switch2/2
  outage/1 -> Bistable2/1
  Bistable2/2 -> Terminator/1
  xy->dq/1(Idq) -> Scope/1, [isdq]
  [xy_dq_delta] -> " control1"/3(delta)
  output/2(isxy) -> isxy/1
  [isxy] -> output/1(is_xy)
  [isxy] -> xy->dq/1(Ixy)
  Isxy/1 -> Switch3/3
  Bistable2/1 -> [outage], NOT/1
  R_choke1/1 -> R_choke2/1
  NOT/1 -> " control1"/Enable
  output/1(m) -> m/1
  [ucxy] -> Sum/2
  R_choke/1 -> Sum/3
  R_choke2/1 -> Sum/4
  Ground/1 -> Bistable2/2
  R_choke3/1 -> Switch2/3
  Sum/1 -> R_choke3/1, Scope4/1
  Selector/1 -> R_choke1/1
  Sum1/1 -> [Dess7]  "Dess4"
  Sum6/1 -> [Hess7]  "Hess4"

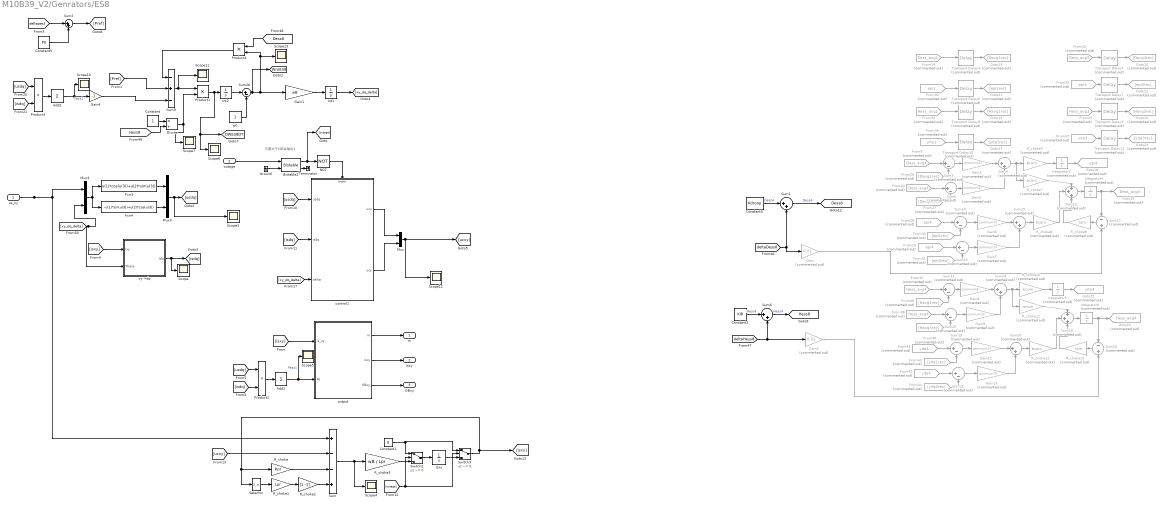
== system M10B39_V2/Genrators/ES8 ==
  note: 只要大于0就会输出1
  us_xy : Inport
  outage : Inport  Port=2
  " control1" : Subsystem
  Add1 : Sum  Inputs=+
  Add2 : Sum  Inputs=+
  Bistable2 : spsBistableLib/Bistable  Qpriority=Set  ic=0  Ts=0
      settings: LibrarySourceBlock=sps_lib/Control/Bistable
  Constant : Constant
  Constant1 : Constant  Value=0
  Constant2 : Constant  Value=KIR
  Constant3 : Constant  Value=Kdroop
  Constant5 : Constant  Value=P0
  Divide : Product  Inputs=*/
  Fcn3 : Fcn  Expr=u(1)*cos(u(3))+u(2)*sin(u(3))
  Fcn4 : Fcn  Expr=-u(1)*sin(u(3))+u(2)*cos(u(3))
  From14 : From  Commented=on  GotoTag=Dess_avg1  TagVisibility=global
  From24 : From  Commented=on  GotoTag=Dess_avg4  TagVisibility=global
  From25 : From  Commented=on  GotoTag=Dess_avg3  TagVisibility=global
  From26 : From  Commented=on  GotoTag=Davg1rec
  From27 : From  Commented=on  GotoTag=Davg3rec
  From28 : From  Commented=on  GotoTag=epi4  TagVisibility=global
  From29 : From  Commented=on  GotoTag=epi4  TagVisibility=global
  From30 : From  Commented=on  GotoTag=epi1rec
  From31 : From  Commented=on  GotoTag=epi3rec
  From32 : From  Commented=on  GotoTag=epi1  TagVisibility=global
  From33 : From  Commented=on  GotoTag=epi3  TagVisibility=global
  From34 : From  Commented=on  GotoTag=Hess_avg1  TagVisibility=global
  From35 : From  Commented=on  GotoTag=Hess_avg3  TagVisibility=global
  From36 : From  Commented=on  GotoTag=yita1  TagVisibility=global
  From37 : From  Commented=on  GotoTag=yita3  TagVisibility=global
  From38 : From  Commented=on  GotoTag=Hess_avg4  TagVisibility=global
  From39 : From  Commented=on  GotoTag=Havg1rec
  From40 : From  Commented=on  GotoTag=Havg3rec
  From41 : From  Commented=on  GotoTag=yita4  TagVisibility=global
  From42 : From  Commented=on  GotoTag=yita4  TagVisibility=global
  From43 : From  Commented=on  GotoTag=yita1rec
  From44 : From  Commented=on  GotoTag=yita3rec
  From45 : From  Commented=on  GotoTag=Hess_avg4  TagVisibility=global
  From9 : From  Commented=on  GotoTag=Dess_avg4  TagVisibility=global
  Gain : Gain  Commented=on  Gain=0.01
  Gain1 : Gain  Gain=wB  SaturateOnIntegerOverflow=on  OutDataTypeStr=Inherit: Same as input  ParamDataTypeStr=Inherit: Same as input
  Gain{3,6,8,12} (4 alike) : Gain  Commented=on  Gain=commun(4)
  Gain{5,7,9,13} (4 alike) : Gain  Commented=on  Gain=commun(3)
  Gain2 : Gain  Commented=on  Gain=0.01
  Gain4 : Gain  Gain=-1
  Goto14 : Goto  Commented=on  GotoTag=Havg1rec
  Goto15 : Goto  Commented=on  GotoTag=Havg3rec
  Goto16 : Goto  Commented=on  GotoTag=Dess_avg4  TagVisibility=global
  Goto17 : Goto  Commented=on  GotoTag=yita1rec
  Goto18 : Goto  Commented=on  GotoTag=epi4  TagVisibility=global
  Goto19 : Goto  Commented=on  GotoTag=Davg1rec
  Goto20 : Goto  Commented=on  GotoTag=Davg3rec
  Goto21 : Goto  Commented=on  GotoTag=epi1rec
  Goto22 : Goto  Commented=on  GotoTag=epi3rec
  Goto23 : Goto  Commented=on  GotoTag=yita3rec
  Goto24 : Goto  Commented=on  GotoTag=Hess_avg4  TagVisibility=global
  Goto25 : Goto  Commented=on  GotoTag=yita4  TagVisibility=global
  Ground : Ground
  Int1 : Integrator  InitialCondition=Dels_hvdc
  Int2 : Integrator  InitialCondition=1
  Integrator{3..6} (4 alike) : Integrator  Commented=on
  Isxy : Integrator  InitialCondition=[Is_xA_0 Is_yA_0]
  Mux : Mux  Inputs=2
  Mux3 : Mux  Inputs=2
  Mux4 : Mux  Inputs=2
  NOT : Logic  Operator=NOT  AllPortsSameDT=off  OutDataTypeStr=boolean
  Product1 : Product
  Product2 : Product  RndMeth=Zero
  Product3 : Product  RndMeth=Zero
  Product4 : Product
  R_choke : Gain  Gain=Rpr  SaturateOnIntegerOverflow=on  OutDataTypeStr=Inherit: Same as input  ParamDataTypeStr=Inherit: Same as input
  R_choke1 : Gain  Gain=Lpr  SaturateOnIntegerOverflow=on  OutDataTypeStr=Inherit: Same as input  ParamDataTypeStr=Inherit: Same as input
  R_choke10 : Gain  Commented=on  Gain=-bcom  SaturateOnIntegerOverflow=on  OutDataTypeStr=Inherit: Same as input  ParamDataTypeStr=Inherit: Same as input
  R_choke11 : Gain  Commented=on  Gain=-acom  SaturateOnIntegerOverflow=on  OutDataTypeStr=Inherit: Same as input  ParamDataTypeStr=Inherit: Same as input
  R_choke12 : Gain  Commented=on  Gain=bcom  SaturateOnIntegerOverflow=on  OutDataTypeStr=Inherit: Same as input  ParamDataTypeStr=Inherit: Same as input
  R_choke13 : Gain  Commented=on  Gain=lam  SaturateOnIntegerOverflow=on  OutDataTypeStr=Inherit: Same as input  ParamDataTypeStr=Inherit: Same as input
  R_choke2 : Gain  Gain=[1 -1]  SaturateOnIntegerOverflow=on  OutDataTypeStr=Inherit: Same as input  ParamDataTypeStr=Inherit: Same as input
  R_choke3 : Gain  Gain=wB / Lpr  SaturateOnIntegerOverflow=on  OutDataTypeStr=Inherit: Same as input  ParamDataTypeStr=Inherit: Same as input
  R_choke4 : Gain  Commented=on  Gain=-bcom  SaturateOnIntegerOverflow=on  OutDataTypeStr=Inherit: Same as input  ParamDataTypeStr=Inherit: Same as input
  R_choke7 : Gain  Commented=on  Gain=-acom  SaturateOnIntegerOverflow=on  OutDataTypeStr=Inherit: Same as input  ParamDataTypeStr=Inherit: Same as input
  R_choke8 : Gain  Commented=on  Gain=bcom  SaturateOnIntegerOverflow=on  OutDataTypeStr=Inherit: Same as input  ParamDataTypeStr=Inherit: Same as input
  R_choke9 : Gain  Commented=on  Gain=lam  SaturateOnIntegerOverflow=on  OutDataTypeStr=Inherit: Same as input  ParamDataTypeStr=Inherit: Same as input
  Scope{,3..7,10..13} (10 alike) : Scope
      Scope settings: ActiveDisplayYMinimum=-0.0194  ActiveDisplayYMaximum=0.04689
      Scope10 settings: ActiveDisplayYMinimum=-6.46308  ActiveDisplayYMaximum=-6.45084
      Scope11 settings: ActiveDisplayYMinimum=-0.1125  ActiveDisplayYMaximum=0.0125  DataLoggingVariableName=ScopeData2
      Scope12 settings: ActiveDisplayYMinimum=0.46883  ActiveDisplayYMaximum=1.25548  DataLoggingVariableName=ScopeData3
      Scope13 settings: ActiveDisplayYMinimum=-0.00656  ActiveDisplayYMaximum=0.05904  DataLoggingVariableName=ScopeData4
      Scope3 settings: ActiveDisplayYMinimum=-0.12696  ActiveDisplayYMaximum=1.14248
      Scope4 settings: ActiveDisplayYMinimum=-2.8E-5  ActiveDisplayYMaximum=2.4E-5  DataLoggingVariableName=ScopeData5
      Scope5 settings: ActiveDisplayYMinimum=-0.00823  ActiveDisplayYMaximum=0.07404  DataLoggingVariableName=ScopeData7
      Scope6 settings: ActiveDisplayYMinimum=-4.9E-5  ActiveDisplayYMaximum=-0  DataLoggingVariableName=ScopeData4
      Scope7 settings: ActiveDisplayYMinimum=0.9  ActiveDisplayYMaximum=1.1  DataLoggingVariableName=ScopeData14
  Selector : Selector  InputPortWidth=2  IndexOptions=Index vector (dialog)  Indices=[2 1]  OutputSizes=1
  Sum : Sum  Inputs=+--+  SaturateOnIntegerOverflow=on
  Sum1 : Sum  Inputs=|++  SaturateOnIntegerOverflow=on
  Sum13 : Sum  Commented=on  Inputs=+++  SaturateOnIntegerOverflow=on
  Sum{3,5,14,16,19,21,23,25} (8 alike) : Sum  Commented=on  Inputs=|+-  SaturateOnIntegerOverflow=on
  Sum{4,15,20,24} (4 alike) : Sum  Commented=on  Inputs=|++  SaturateOnIntegerOverflow=on
  Sum17 : Sum  Commented=on  Inputs=-+  SaturateOnIntegerOverflow=on
  Sum18 : Sum  Commented=on  Inputs=+++  SaturateOnIntegerOverflow=on
  Sum2 : Sum  Inputs=|++
  Sum22 : Sum  Commented=on  Inputs=-+  SaturateOnIntegerOverflow=on
  Sum26 : Sum  Inputs=|+-  SaturateOnIntegerOverflow=on
  Sum6 : Sum  Inputs=|++  SaturateOnIntegerOverflow=on
  Sum9 : Sum  Inputs=-+-  SaturateOnIntegerOverflow=on
  Switch2 : Switch  Criteria=u2 ~= 0  Threshold=0.5  InputSameDT=off
  Switch3 : Switch  Criteria=u2 ~= 0  Threshold=0.5  InputSameDT=off
  Terminator : Terminator
  Transport Delay{4,6,8,10} (4 alike) : TransportDelay  Commented=on  DelayTime=DataDelay(1,1)
  Transport Delay{5,7,9,11} (4 alike) : TransportDelay  Commented=on  DelayTime=DataDelay(3,2)
  output : Subsystem
  w0 : Constant
  xy->dq : Subsystem
  m : Outport
  isxy : Outport  Port=2
  GBxy : Outport  Port=3
  tag scope: DWES8DT=global, Dess8=global, Hess8=global, WreES8=global
  wires:
  Gain13/1 -> Sum20/2
  Sum21/1 -> Gain13/1
  Sum19/1 -> Gain12/1
  Gain12/1 -> Sum20/1
  Sum25/1 -> Gain9/1
  Gain9/1 -> Sum24/2
  Gain8/1 -> Sum24/1
  Sum23/1 -> Gain8/1
  Gain7/1 -> Sum15/2
  Sum16/1 -> Gain7/1
  Sum14/1 -> Gain6/1
  Gain6/1 -> Sum15/1
  Gain5/1 -> Sum4/2
  Sum5/1 -> Gain5/1
  Gain3/1 -> Sum4/1
  Sum3/1 -> Gain3/1
  From37/1 -> Transport Delay11/1
  From35/1 -> Transport Delay9/1
  From33/1 -> Transport Delay7/1
  From25/1 -> Transport Delay5/1
  From36/1 -> Transport Delay10/1
  From34/1 -> Transport Delay8/1
  From32/1 -> Transport Delay6/1
  From14/1 -> Transport Delay4/1
  Gain2/1 -> Sum22/2
  Gain/1 -> Sum17/2
  [deltaHess8] -> Sum6/2, Gain2/1
  Integrator5/1 -> Goto25/1
  From43/1 -> Sum19/2
  Integrator6/1 -> Goto24/1, Sum22/1
  From9/1 -> Sum3/1
  From27/1 -> Sum5/2
  R_choke11/1 -> Sum18/1
  From44/1 -> Sum21/2
  Sum4/1 -> R_choke4/1, R_choke7/1
  From41/1 -> Sum19/1
  R_choke13/1 -> Sum18/3
  Sum22/1 -> R_choke13/1
  From38/1 -> Sum25/1
  R_choke12/1 -> Sum18/2
  Sum18/1 -> Integrator6/1
  R_choke7/1 -> Sum13/1
  From24/1 -> Sum5/1
  From28/1 -> Sum14/1
  R_choke8/1 -> Sum13/2
  From42/1 -> Sum21/1
  R_choke10/1 -> Integrator5/1
  From45/1 -> Sum23/1
  Transport Delay11/1 -> Goto23/1
  Transport Delay9/1 -> Goto15/1
  From40/1 -> Sum25/2
  Transport Delay10/1 -> Goto17/1
  Sum13/1 -> Integrator4/1
  Transport Delay6/1 -> Goto21/1
  Sum17/1 -> R_choke9/1
  Transport Delay8/1 -> Goto14/1
  From39/1 -> Sum23/2
  Transport Delay7/1 -> Goto22/1
  R_choke4/1 -> Integrator3/1
  Transport Delay5/1 -> Goto20/1
  Transport Delay4/1 -> Goto19/1
  From26/1 -> Sum3/2
  Sum15/1 -> R_choke8/1
  Integrator3/1 -> Goto18/1
  Sum24/1 -> R_choke10/1, R_choke11/1
  Constant3/1 -> Sum1/1  "Dess4"
  From29/1 -> Sum16/1
  Constant2/1 -> Sum6/1  "Hess4"
  Sum20/1 -> R_choke12/1
  R_choke9/1 -> Sum13/3
  [deltaDess8] -> Gain/1, Sum1/2
  From31/1 -> Sum16/2
  From30/1 -> Sum14/2
  Integrator4/1 -> Goto16/1, Sum17/1
  Gain1/1 -> Int1/1
  [Dess8] -> Product4/1
  Product3/1 -> Add2/1
  [isdq] -> Product3/2
  [usdq] -> Product3/1
  Add2/1 -> Scope10/1, Gain4/1  "Pess1"
  Int1/1 -> [xy_dq_delta]
  Product4/1 -> Sum9/1
  Gain4/1 -> Sum9/3
  Mux3/1 -> [usdq], Scope3/1
  [xy_dq_delta] -> xy->dq/2(Theta), Mux4/2
  Mux4/1 -> Fcn4/1, Fcn3/1
  Fcn4/1 -> Mux3/2
  Fcn3/1 -> Mux3/1
  us_xy/1 -> Sum/1, Mux4/1
  [Hess8] -> Divide/2
  Divide/1 -> Scope7/1, Product1/2
  Constant/1 -> Divide/1
  Sum9/1 -> Scope11/1, Product1/1
  w0/1 -> Sum26/2
  Int2/1 -> Sum26/1
  Sum26/1 -> Product4/2, Scope13/1, Gain1/1, [WreES8]
  Product1/1 -> Int2/1, [DWES8DT], Scope6/1
  [isdq] -> Product2/2
  Product2/1 -> Add1/1
  Add1/1 -> output/2(Pe), Scope5/1  "Pess1"
  [usdq] -> Product2/1
  " control1"/2(ucy) -> Mux/2
  Constant1/1 -> Switch3/1, Switch2/1
  output/3(GBxy) -> GBxy/1
  [usdq] -> " control1"/1(usdq)
  Mux/1 -> [ucxy], Scope12/1
  Switch3/1 -> [isxy], Selector/1, R_choke/1
  Switch2/1 -> Isxy/1
  " control1"/1(ucx) -> Mux/1
  [isdq] -> " control1"/2(isdq)
  [outage] -> Switch3/2, Switch2/2
  outage/1 -> Bistable2/1
  Bistable2/2 -> Terminator/1
  xy->dq/1(Idq) -> Scope/1, [isdq]
  [xy_dq_delta] -> " control1"/3(delta)
  output/2(isxy) -> isxy/1
  [isxy] -> output/1(is_xy)
  [isxy] -> xy->dq/1(Ixy)
  Isxy/1 -> Switch3/3
  Bistable2/1 -> [outage], NOT/1
  R_choke1/1 -> R_choke2/1
  NOT/1 -> " control1"/Enable
  output/1(m) -> m/1
  [ucxy] -> Sum/2
  R_choke/1 -> Sum/3
  R_choke2/1 -> Sum/4
  Ground/1 -> Bistable2/2
  R_choke3/1 -> Switch2/3
  Sum/1 -> R_choke3/1, Scope4/1
  Selector/1 -> R_choke1/1
  Sum1/1 -> [Dess8]  "Dess4"
  Sum6/1 -> [Hess8]  "Hess4"
  Constant5/1 -> Sum2/2
  Sum2/1 -> [Pref]
  [deltapes3] -> Sum2/1
  [Pref] -> Sum9/2

== system M10B39_V2/Genrators/Generator10 ==
  Vgxy : Inport
  Trip : Inport  Port=2
  Bistable2 : spsBistableLib/Bistable  Qpriority=Set  ic=0  Ts=0
      settings: LibrarySourceBlock=sps_lib/Control/Bistable
  Constant : Constant  Value=[0,0,0,0]
  Excitation System ST1A1 : Subsystem
  Governor : Subsystem
  Ground : Ground
  "Machine Equations " : Subsystem
  Mechanical DE : Subsystem
  Output : Subsystem
  PSS1 : Subsystem
  Scope{,1..3,5} (5 alike) : Scope
      Scope settings: ActiveDisplayYMinimum=-0.52997  ActiveDisplayYMaximum=12.90306  DataLoggingVariableName=ScopeData3
      Scope1 settings: ActiveDisplayYMinimum=7.63415  ActiveDisplayYMaximum=7.96859  DataLoggingVariableName=ScopeData2
      Scope2 settings: TimeSpan=10  ActiveDisplayYMinimum=-0.0003  ActiveDisplayYMaximum=0.0004  DataLoggingVariableName=ScopeData22
      Scope3 settings: TimeSpan=10  ActiveDisplayYMinimum=0.54572  ActiveDisplayYMaximum=0.55101  DataLoggingVariableName=ScopeData23
      Scope5 settings: TimeSpan=10  ActiveDisplayYMinimum=0.15  ActiveDisplayYMaximum=0.65  DataLoggingVariableName=ScopeData10
  Switch4 : Switch  Criteria=u2 ~= 0  Threshold=0.5  InputSameDT=off
  Terminator : Terminator
  pu->pu : Gain  Gain=SgenB./SgridB
  pu->pu1 : Gain  Gain=SgenB./SgridB
  m : Outport
  Igxy1 : Outport  Port=2
  GBxy : Outport  Port=3
  wires:
  pu->pu1/1 -> [GBxy]
  pu->pu/1 -> [Igxy1]
  "Machine Equations "/3(GBxy) -> Switch4/3
  Constant/1 -> Switch4/1
  Switch4/1 -> pu->pu1/1
  [Trip] -> Switch4/2
  [Trip] -> PSS1/2(Trip)
  [Trip] -> Governor/2(Trip)
  [Trip] -> Mechanical DE/3(Trip)
  [Trip] -> Excitation System ST1A1/2(Trip)
  [Trip] -> "Machine Equations "/4(Trip)
  Bistable2/2 -> Terminator/1
  Trip/1 -> Bistable2/1
  Ground/1 -> Bistable2/2
  Bistable2/1 -> [Trip]
  [Vg] -> Output/6(Vg)
  Output/1(m) -> m/1
  Output/3(GBxy) -> GBxy/1
  Output/2(Igxy1) -> Igxy1/1
  [Igxy1] -> Output/1(Igxy1in)
  [GBxy] -> Output/2(GBxyin)
  [delta] -> Output/3(deltain)
  [f] -> Output/5(fin)
  [Pe] -> Output/4(Pein)
  Mechanical DE/1(delta) -> "Machine Equations "/1(delta), [delta], Scope/1
  Governor/1(dPm) -> Scope3/1, Mechanical DE/2(dPm)
  PSS1/1(Upss) -> Scope2/1, Excitation System ST1A1/1(Upss)
  Mechanical DE/2(w) -> [f], PSS1/1(w), Governor/1(w)
  "Machine Equations "/2(Igxy1) -> pu->pu/1
  Vgxy/1 -> "Machine Equations "/2(Vgxy)
  "Machine Equations "/4(Vg) -> [Vg], Excitation System ST1A1/3(Vg)
  "Machine Equations "/1(Pe) -> [Pe], Mechanical DE/1(Pe), Scope1/1
  Excitation System ST1A1/1(Ef) -> "Machine Equations "/3(Ef), Scope5/1
